simulink model "model_5LinkWalk_NODS_soft_ground"  (R2022b)
settings: Solver=VariableStepAuto  StartTime=0.0  StopTime=Tf  FixedStep=1e-5  MaxStep=1e-3  RelTol=1e-12  AbsTol=1e-8
values from neighbouring files (symbols this model uses):
  gains = [K_p,K_d,K_p,K_d,K_p,K_d,K_p,K_d,K_p,K_d]    [main_soft_ground.m]
  init_flag = [-1; 0; ocl_traj.x_sw(1); init_t_mode_change; alpha_ref(1); 0; y_g_curr]    [main_soft_ground.m]
  Initial_state = [q0;dq0]    [main_soft_ground.m]
  joint_angles_ref = [ocl_traj.time, ocl_traj.simout, alpha_ref]    [main_soft_ground.m]
  landing_ref = [landing_traj.time, landing_traj.simout, alpha_ref_landing]    [main_soft_ground.m]
  param = [ ... (first row only)    [main_soft_ground.m]
  sample_time = time(2) - time(1)    [animation_floating.m]    (also in main_soft_ground.m = 0.001)
undefined symbols (not defined in the file or in its folder): uneven_terrain
libraries: simulink x2
(part 1 of 2)
settings Model: SimulationMode=accelerator  VariantFading=off  Creator=yamakita_lab  LastModifiedBy=mmpel
settings SolverCC: AutoScaleAbsTol=off  AlgebraicLoopSolver=TrustRegion
settings DataIOCC: ReturnWorkspaceOutputs=off
settings DebuggingCC: ParameterPrecisionLossMsg=none  UnconnectedInputMsg=warning  UnconnectedOutputMsg=warning  UnconnectedLineMsg=warning  SFMachineParentedDataDiag=warning  ArithmeticOperatorsInVariantConditions=warning
settings ModelReferenceCC: EnableRefExpFcnMdlSchedulingChecks=on
settings SFSimCC: SimUseLocalCustomCode=off  CustomCodeUndefinedFunction=UseInterfaceOnly
settings RTWCC: RTWUseLocalCustomCode=off  DLArmComputeVersion=19.05

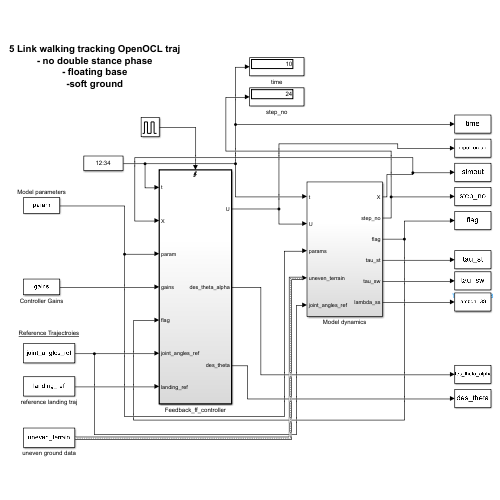
[thumbnail: Simulink's stored preview of the top-level diagram]
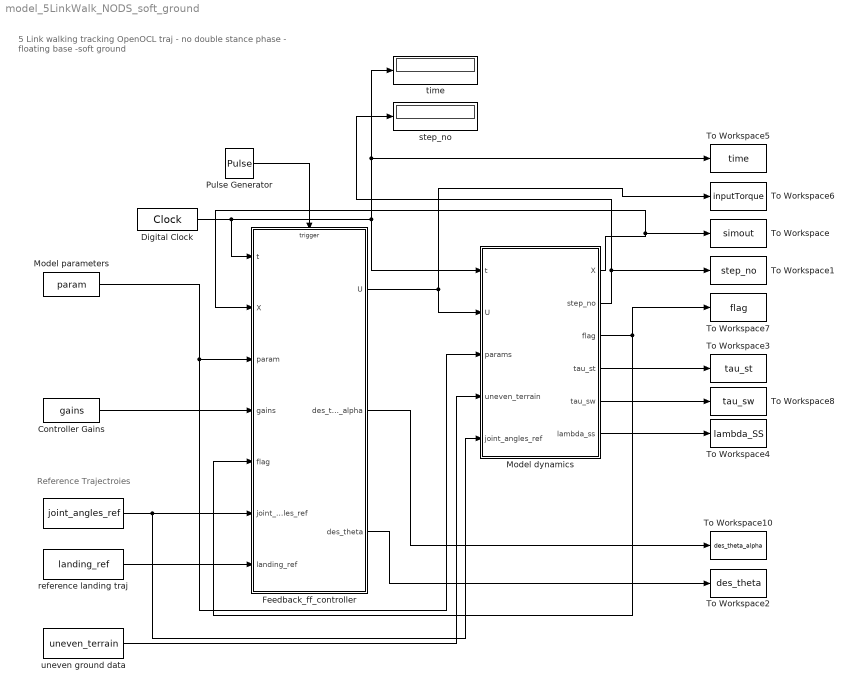
== system model_5LinkWalk_NODS_soft_ground ==
  note: Reference Trajectroies
  note: 5 Link walking tracking OpenOCL traj
      | - no double stance phase
      | - floating base
      | -soft ground
  " " : Constant  Value=joint_angles_ref
  Controller Gains : Constant  Value=gains
  Digital Clock : DigitalClock  SampleTime=1e-4
  Feedback_ff_controller : Subsystem  TreatAsAtomicUnit=on
  Model dynamics : Subsystem
  Model parameters : Constant  Value=param  OutDataTypeStr=double
  Pulse Generator : DiscretePulseGenerator  PulseType=Time based  Period=5e-4  PulseWidth=5
  To Workspace : ToWorkspace  VariableName=simout  SampleTime=sample_time
  To Workspace1 : ToWorkspace  VariableName=step_no  SampleTime=sample_time
  To Workspace10 : ToWorkspace  VariableName=des_theta_alpha  SampleTime=sample_time
  To Workspace2 : ToWorkspace  VariableName=des_theta  SampleTime=sample_time
  To Workspace3 : ToWorkspace  VariableName=tau_st  SampleTime=sample_time
  To Workspace4 : ToWorkspace  VariableName=lambda_SS  SampleTime=sample_time
  To Workspace5 : ToWorkspace  VariableName=time  SampleTime=sample_time
  To Workspace6 : ToWorkspace  VariableName=inputTorque  SampleTime=sample_time
  To Workspace7 : ToWorkspace  VariableName=flag  SampleTime=sample_time
  To Workspace8 : ToWorkspace  VariableName=tau_sw  SampleTime=sample_time
  reference landing traj : Constant  Value=landing_ref
  step_no : Display
  time : Display
  uneven ground data : Constant  Value=uneven_terrain  OutDataTypeStr=Bus: uneven_terrain_bus
  wires:
  Feedback_ff_controller/1(U) -> Model dynamics/2(U), To Workspace6/1
  Model dynamics/1(X) -> To Workspace/1, Feedback_ff_controller/2(X)
  Digital Clock/1 -> time/1, To Workspace5/1, Model dynamics/1(t), Feedback_ff_controller/1(t)
  Model dynamics/2(step_no) -> step_no/1, To Workspace1/1
  Model parameters/1 -> Model dynamics/3(params), Feedback_ff_controller/3(param)
  Controller Gains/1 -> Feedback_ff_controller/4(gains)
  Model dynamics/3(flag) -> Feedback_ff_controller/5(flag), To Workspace7/1
  " "/1 -> Model dynamics/5(joint_angles_ref), Feedback_ff_controller/6(joint_angles_ref)
  Pulse Generator/1 -> Feedback_ff_controller/Trigger
  Model dynamics/4(tau_st) -> To Workspace3/1
  Model dynamics/5(tau_sw) -> To Workspace8/1
  Feedback_ff_controller/2(des_theta_alpha) -> To Workspace10/1
  Feedback_ff_controller/3(des_theta) -> To Workspace2/1
  uneven ground data/1 -> Model dynamics/4(uneven_terrain)
  reference landing traj/1 -> Feedback_ff_controller/7(landing_ref)
  Model dynamics/6(lambda_ss) -> To Workspace4/1

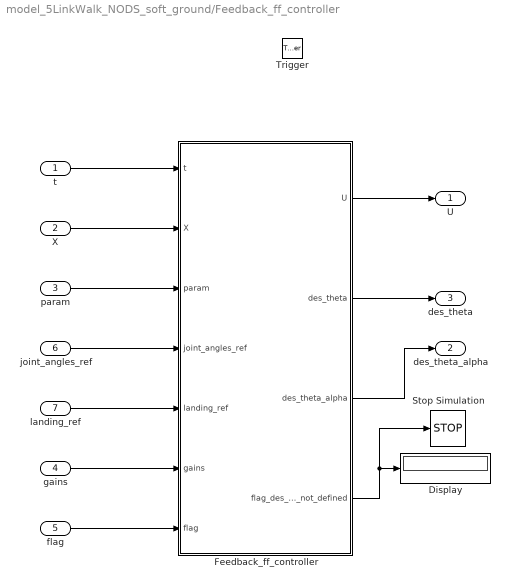
== system model_5LinkWalk_NODS_soft_ground/Feedback_ff_controller ==
  t : Inport
  X : Inport  Port=2
  param : Inport  Port=3
  gains : Inport  Port=4
  flag : Inport  Port=5
  joint_angles_ref : Inport  Port=6
  landing_ref : Inport  Port=7
  Trigger : TriggerPort  VariantControl=Variant  PortDimensions=1
  Display : Display
  Feedback_ff_controller : MATLAB Function  TreatAsAtomicUnit=on
  Stop Simulation : Stop
  U : Outport  VectorParamsAs1DForOutWhenUnconnected=off
  des_theta_alpha : Outport  Port=2  InitialOutput=[0;0;0;0;0; 0;0;0;0;0; 0]  VectorParamsAs1DForOutWhenUnconnected=off
  des_theta : Outport  Port=3  InitialOutput=[0;0;0;0;0; 0;0;0;0;0]  VectorParamsAs1DForOutWhenUnconnected=off
  wires:
  Feedback_ff_controller/1(U) -> U/1
  t/1 -> Feedback_ff_controller/1(t)
  X/1 -> Feedback_ff_controller/2(X)
  param/1 -> Feedback_ff_controller/3(param)
  gains/1 -> Feedback_ff_controller/6(gains)
  flag/1 -> Feedback_ff_controller/7(flag)
  joint_angles_ref/1 -> Feedback_ff_controller/4(joint_angles_ref)
  Feedback_ff_controller/3(des_theta_alpha) -> des_theta_alpha/1
  landing_ref/1 -> Feedback_ff_controller/5(landing_ref)
  Feedback_ff_controller/4(flag_des_theta_not_defined) -> Stop Simulation/1, Display/1
  Feedback_ff_controller/2(des_theta) -> des_theta/1

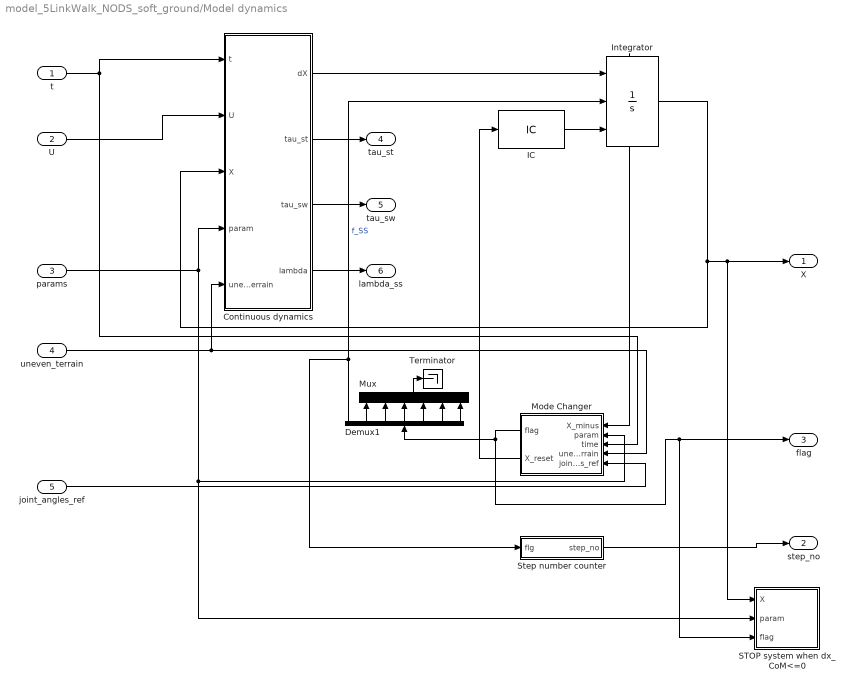
== system model_5LinkWalk_NODS_soft_ground/Model dynamics ==
  t : Inport
  U : Inport  Port=2
  params : Inport  Port=3
  uneven_terrain : Inport  Port=4
  joint_angles_ref : Inport  Port=5
  Continuous dynamics : MATLAB Function  TreatAsAtomicUnit=on
  Demux1 : Demux  Outputs=7
  IC : InitialCondition  Value=Initial_state
  Integrator : Integrator  ExternalReset=rising  InitialConditionSource=external  ShowStatePort=on
  Mode Changer : Subsystem
  Mux : Mux  Inputs=6
  STOP system when dx_CoM<=0 : Subsystem
  Step number counter : Subsystem
  Terminator : Terminator
  X : Outport  VectorParamsAs1DForOutWhenUnconnected=off
  step_no : Outport  Port=2  VectorParamsAs1DForOutWhenUnconnected=off
  flag : Outport  Port=3
  tau_st : Outport  Port=4  VectorParamsAs1DForOutWhenUnconnected=off
  tau_sw : Outport  Port=5  VectorParamsAs1DForOutWhenUnconnected=off
  lambda_ss : Outport  Port=6  VectorParamsAs1DForOutWhenUnconnected=off
  wires:
  IC/1 -> Integrator/3
  Integrator/State -> Mode Changer/1(X_minus)
  Continuous dynamics/1(dX) -> Integrator/1
  params/1 -> Continuous dynamics/4(param), STOP system when dx_CoM<=0/2(param), Mode Changer/2("param ")
  U/1 -> Continuous dynamics/2(U)
  t/1 -> Continuous dynamics/1(t), Mode Changer/3(time)
  Integrator/1 -> STOP system when dx_CoM<=0/1(X), X/1, Continuous dynamics/3(X)
  Mode Changer/2(X_reset) -> IC/1
  Mode Changer/1(flag) -> STOP system when dx_CoM<=0/3(flag), flag/1, Demux1/1
  Demux1/1 -> Integrator/2, Step number counter/1(flg)  "f_SS"
  Step number counter/1(step_no) -> step_no/1
  Continuous dynamics/2(tau_st) -> tau_st/1
  Continuous dynamics/3(tau_sw) -> tau_sw/1
  Demux1/2 -> Mux/1
  Demux1/3 -> Mux/2
  Demux1/4 -> Mux/3
  Demux1/5 -> Mux/4
  Demux1/6 -> Mux/5
  Mux/1 -> Terminator/1
  uneven_terrain/1 -> Continuous dynamics/5(uneven_terrain), Mode Changer/4(uneven_terrain)
  Demux1/7 -> Mux/6
  joint_angles_ref/1 -> Mode Changer/5(joint_angles_ref)
  Continuous dynamics/4(lambda) -> lambda_ss/1

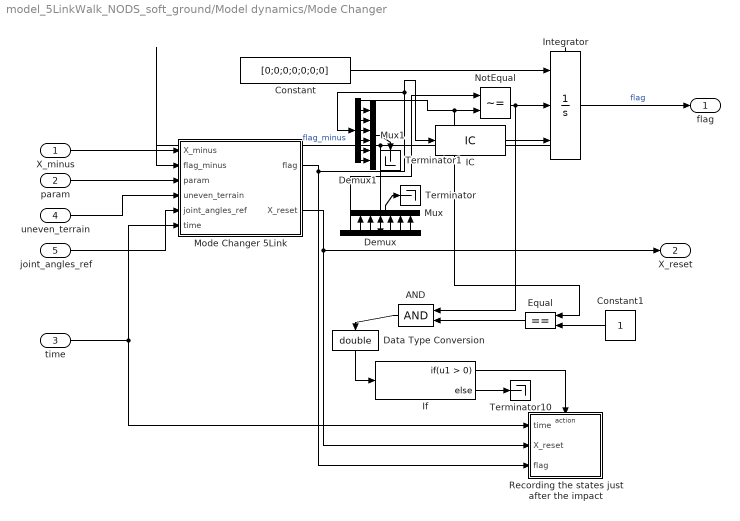
== system model_5LinkWalk_NODS_soft_ground/Model dynamics/Mode Changer ==
  X_minus : Inport
  "param " : Inport  Port=2
  time : Inport  Port=3
  uneven_terrain : Inport  Port=4
  joint_angles_ref : Inport  Port=5
  AND : Logic  IconShape=distinctive  AllPortsSameDT=off  OutDataTypeStr=boolean
  Constant : Constant  Value=[0;0;0;0;0;0;0]
  Constant1 : Constant
  Data Type Conversion : DataTypeConversion  OutDataTypeStr=double  SaturateOnIntegerOverflow=off  RndMeth=Floor
  Demux : Demux  Outputs=7
  Demux1 : Demux  Outputs=7
  Equal : RelationalOperator  Operator===  OutDataTypeStr=boolean  RndMeth=Simplest  InputSameDT=off
  IC : InitialCondition  Value=init_flag
  If : If
  Integrator : Integrator  ExternalReset=rising  InitialConditionSource=external  ShowStatePort=on
  Mode Changer 5Link : MATLAB Function  TreatAsAtomicUnit=on
  Mux : Mux  Inputs=6
  Mux1 : Mux  Inputs=6
  NotEqual : RelationalOperator  Operator=~=  OutDataTypeStr=boolean  RndMeth=Simplest  InputSameDT=off
  Recording the states just after the impact : Subsystem  TreatAsAtomicUnit=on
  Terminator : Terminator
  Terminator1 : Terminator
  Terminator10 : Terminator
  flag : Outport  VectorParamsAs1DForOutWhenUnconnected=off
  X_reset : Outport  Port=2  VectorParamsAs1DForOutWhenUnconnected=off
  wires:
  X_minus/1 -> Mode Changer 5Link/1(X_minus)
  IC/1 -> Integrator/3
  Integrator/State -> Mode Changer 5Link/2(flag_minus), Demux/1  "flag_minus"
  "param "/1 -> Mode Changer 5Link/3(param)
  Mode Changer 5Link/1(flag) -> Demux1/1, IC/1, Recording the states just after the impact/3(flag)
  Constant/1 -> Integrator/1
  NotEqual/1 -> AND/1, Integrator/2
  Integrator/1 -> flag/1  "flag"
  Mode Changer 5Link/2(X_reset) -> Recording the states just after the impact/2(X_reset), X_reset/1
  Demux/1 -> NotEqual/1
  time/1 -> Mode Changer 5Link/6(time), Recording the states just after the impact/1(time)
  Demux1/1 -> Equal/1, NotEqual/2
  If/1 -> Recording the states just after the impact/Action
  If/2 -> Terminator10/1
  Data Type Conversion/1 -> If/1
  AND/1 -> Data Type Conversion/1
  Equal/1 -> AND/2
  Constant1/1 -> Equal/2
  uneven_terrain/1 -> Mode Changer 5Link/4(uneven_terrain)
  Demux/2 -> Mux/1
  Demux/3 -> Mux/2
  Demux/4 -> Mux/3
  Demux/5 -> Mux/4
  Demux/6 -> Mux/5
  Demux/7 -> Mux/6
  Mux/1 -> Terminator/1
  Demux1/2 -> Mux1/1
  Demux1/3 -> Mux1/2
  Demux1/4 -> Mux1/3
  Demux1/5 -> Mux1/4
  Demux1/6 -> Mux1/5
  Demux1/7 -> Mux1/6
  Mux1/1 -> Terminator1/1
  joint_angles_ref/1 -> Mode Changer 5Link/5(joint_angles_ref)

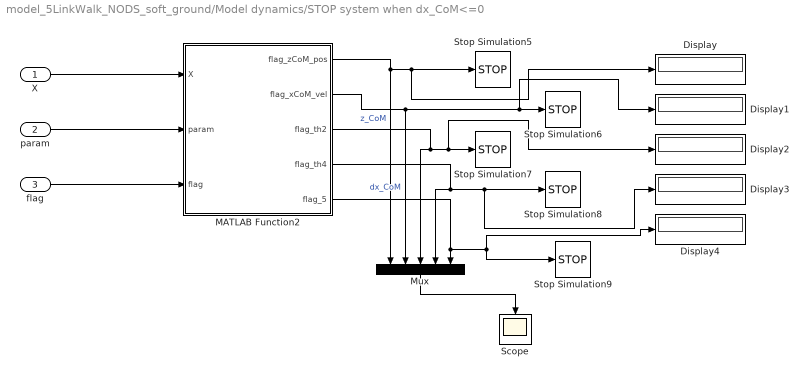
== system model_5LinkWalk_NODS_soft_ground/Model dynamics/STOP system when dx_CoM<=0 ==
  X : Inport
  param : Inport  Port=2
  flag : Inport  Port=3
  Display{,1..4} (5 alike) : Display
  MATLAB Function2 : MATLAB Function  TreatAsAtomicUnit=on
  Mux : Mux  Inputs=5
  Scope : Scope
  Stop Simulation{5..9} (5 alike) : Stop
  wires:
  X/1 -> MATLAB Function2/1(X)
  param/1 -> MATLAB Function2/2(param)
  flag/1 -> MATLAB Function2/3(flag)
  MATLAB Function2/1(flag_zCoM_pos) -> Mux/1, Display/1, Stop Simulation5/1  "z_CoM"
  MATLAB Function2/2(flag_xCoM_vel) -> Display1/1, Stop Simulation6/1, Mux/2  "dx_CoM"
  MATLAB Function2/4(flag_th4) -> Mux/4, Display3/1, Stop Simulation8/1
  Mux/1 -> Scope/1
  MATLAB Function2/3(flag_th2) -> Display2/1, Stop Simulation7/1, Mux/3
  MATLAB Function2/5(flag_5) -> Display4/1, Stop Simulation9/1, Mux/5

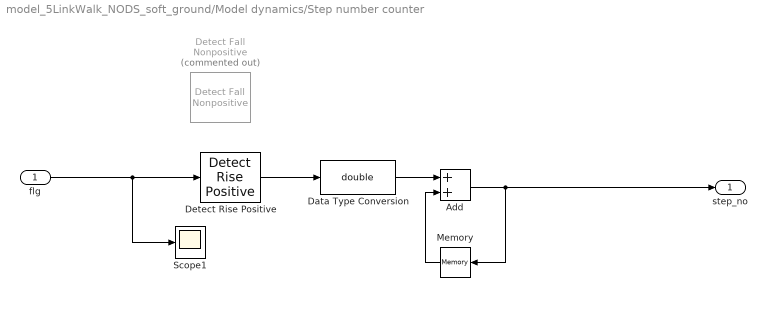
== system model_5LinkWalk_NODS_soft_ground/Model dynamics/Step number counter ==
  flg : Inport  SampleTime=sample_time
  Add : Sum
  Data Type Conversion : DataTypeConversion  OutDataTypeStr=double  SaturateOnIntegerOverflow=off  RndMeth=Floor
  Detect Fall Nonpositive : simulink/Logic and Bit Operations/Detect Fall Nonpositive  Commented=on  vinit=1  OutDataTypeStr=boolean
  Detect Rise Positive : simulink/Logic and Bit Operations/Detect Rise Positive  vinit=-1  OutDataTypeStr=boolean
  Memory : Memory  InheritSampleTime=on
  Scope1 : Scope
  step_no : Outport  VectorParamsAs1DForOutWhenUnconnected=off
  wires:
  Add/1 -> step_no/1, Memory/1
  Memory/1 -> Add/2
  flg/1 -> Detect Rise Positive/1, Scope1/1
  Data Type Conversion/1 -> Add/1
  Detect Rise Positive/1 -> Data Type Conversion/1

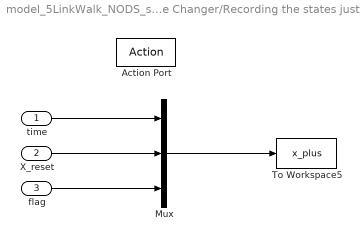
== system model_5LinkWalk_NODS_soft_ground/Model dynamics/Mode Changer/Recording the states just after the impact ==
  time : Inport
  X_reset : Inport  Port=2
  flag : Inport  Port=3
  Action Port : ActionPort  ActionPortLabel=if(u1 > 0)
  Mux : Mux  Inputs=3
  To Workspace5 : ToWorkspace  VariableName=x_plus  SampleTime=-1
  wires:
  time/1 -> Mux/1
  X_reset/1 -> Mux/2
  flag/1 -> Mux/3
  Mux/1 -> To Workspace5/1

== matlab function model_5LinkWalk_NODS_soft_ground/Model dynamics/Continuous dynamics ==
  data: t input; U input; dX output; X input; param input; tau_st output; tau_sw output; lambda output; uneven_terrain input
function [dX, tau_st, tau_sw, lambda] = fcn(t, U, X, param, uneven_terrain)

%% variables
x_st = X(1);
y_st = X(2);
th1 = X(3);
th2 = X(4);
th3 = X(5);
th4 = X(6);
th5 = X(7);

dx_st = X(8);
dy_st = X(9);
dth1 = X(10);
dth2 = X(11);
dth3 = X(12);
dth4 = X(13);
dth5 = X(14);

q = [x_st; y_st; th1; th2; th3; th4; th5];
dq = [dx_st; dy_st; dth1; dth2; dth3; dth4; dth5];

%% parameters

m1 = param(1);
m2 = param(2);
m3 = m2;
m4 = m1;
m5 = param(3);

l1 = param(4);
l2 = param(5);
l5 = param(6);
l3 = l2;
l4 = l1;

gravi = param(7);
I1 = param(8);
I2 = param(9);
I5 = param(10);
I3 = I1;
I4 = I2;

r_k = param(11);
r_h = param(12);
k_ba = param(13);
phi_h0 = param(14);
phi_k0 = param(15);

% ground parameters
k_ground = param(16);
d_ground = param(17);

%% ground height below the stance foot
x_ground = uneven_terrain.track_start:uneven_terrain.dist_step_size:uneven_terrain.track_end;
y_ground = uneven_terrain.y_g_curr;
y_ground_curr = interp1(x_ground, y_ground, x_st);

%% flags
% f_SS = flag(1); % indicates which stance phase it is
% foot = flag(2); % location of the stance foot
% foot_prev = flag(3); % previous location of the stance foot

%% Inertia Matrix
MM = [m1 + m2 + m3 + m4 + m5, 0, - (m3*(2*l2*sin(th1 + th2) + 2*l1*sin(th1) + l3*sin(th1 + th2 + th3)))/2 - (m5*(2*l2*sin(th1 + th2) + 2*l1*sin(th1) + l5*sin(th1 + th2 + th5)))/2 - (m2*(l2*sin(th1 + th2) + 2*l1*sin(th1)))/2 - (m4*(l4*sin(th1 + th2 + th3 + th4) + 2*l2*sin(th1 + th2) + 2*l1*sin(th1) + 2*l3*sin(th1 + th2 + th3)))/2 - (l1*m1*sin(th1))/2, - (m4*(l4*sin(th1 + th2 + th3 + th4) + 2*l2*sin(th1 + th2) + 2*l3*sin(th1 + th2 + th3)))/2 - (m3*(2*l2*sin(th1 + th2) + l3*sin(th1 + th2 + th3)))/2 - (m5*(2*l2*sin(th1 + th2) + l5*sin(th1 + th2 + th5)))/2 - (l2*m2*sin(th1 + th2))/2, - (m4*(l4*sin(th1 + th2 + th3 + th4) + 2*l3*sin(th1 + th2 + th3)))/2 - (l3*m3*sin(th1 + th2 + th3))/2, -(l4*m4*sin(th1 + th2 + th3 + th4))/2, -(l5*m5*sin(th1 + th2 + th5))/2; 0, m1 + m2 + m3 + m4 + m5, (m3*(2*l2*cos(th1 + th2) + 2*l1*cos(th1) + l3*cos(th1 + th2 + th3)))/2 + (m5*(2*l2*cos(th1 + th2) + 2*l1*cos(th1) + l5*cos(th1 + th2 + th5)))/2 + (m2*(l2*cos(th1 + th2) + 2*l1*cos(th1)))/2 + (m4*(l4*cos(th1 + th2 + th3 + th4) + 2*l2*cos(th1 + th2) + 2*l1*cos(th1) + 2*l3*cos(th1 + th2 + th3)))/2 + (l1*m1*cos(th1))/2, (m3*(2*l2*cos(th1 + th2) + l3*cos(th1 + th2 + th3)))/2 + (m5*(2*l2*cos(th1 + th2) + l5*cos(th1 + th2 + th5)))/2 + (m4*(l4*cos(th1 + th2 + th3 + th4) + 2*l2*cos(th1 + th2) + 2*l3*cos(th1 + th2 + th3)))/2 + (l2*m2*cos(th1 + th2))/2, (m4*(l4*cos(th1 + th2 + th3 + th4) + 2*l3*cos(th1 + th2 + th3)))/2 + (l3*m3*cos(th1 + th2 + th3))/2, (l4*m4*cos(th1 + th2 + th3 + th4))/2, (l5*m5*cos(th1 + th2 + th5))/2; - (m3*(2*l2*sin(th1 + th2) + 2*l1*sin(th1) + l3*sin(th1 + th2 + th3)))/2 - (m5*(2*l2*sin(th1 + th2) + 2*l1*sin(th1) + l5*sin(th1 + th2 + th5)))/2 - (m2*(l2*sin(th1 + th2) + 2*l1*sin(th1)))/2 - (m4*(l4*sin(th1 + th2 + th3 + th4) + 2*l2*sin(th1 + th2) + 2*l1*sin(th1) + 2*l3*sin(th1 + th2 + th3)))/2 - (l1*m1*sin(th1))/2, (m3*(2*l2*cos(th1 + th2) + 2*l1*cos(th1) + l3*cos(th1 + th2 + th3)))/2 + (m5*(2*l2*cos(th1 + th2) + 2*l1*cos(th1) + l5*cos(th1 + th2 + th5)))/2 + (m2*(l2*cos(th1 + th2) + 2*l1*cos(th1)))/2 + (m4*(l4*cos(th1 + th2 + th3 + th4) + 2*l2*cos(th1 + th2) + 2*l1*cos(th1) + 2*l3*cos(th1 + th2 + th3)))/2 + (l1*m1*cos(th1))/2, I1 + I2 + I3 + I4 + I5 + (l1^2*m1)/4 + l1^2*m2 + l1^2*m3 + (l2^2*m2)/4 + l1^2*m4 + l2^2*m3 + l1^2*m5 + l2^2*m4 + (l3^2*m3)/4 + l2^2*m5 + l3^2*m4 + (l4^2*m4)/4 + (l5^2*m5)/4 + l1*l3*m3*cos(th2 + th3) + 2*l1*l3*m4*cos(th2 + th3) + l2*l4*m4*cos(th3 + th4) + l1*l5*m5*cos(th2 + th5) + l1*l2*m2*cos(th2) + 2*l1*l2*m3*cos(th2) + 2*l1*l2*m4*cos(th2) + 2*l1*l2*m5*cos(th2) + l2*l3*m3*cos(th3) + 2*l2*l3*m4*cos(th3) + l3*l4*m4*cos(th4) + l2*l5*m5*cos(th5) + l1*l4*m4*cos(th2 + th3 + th4), I2 + I3 + I4 + I5 + (l2^2*m2)/4 + l2^2*m3 + l2^2*m4 + (l3^2*m3)/4 + l2^2*m5 + l3^2*m4 + (l4^2*m4)/4 + (l5^2*m5)/4 + (l1*l3*m3*cos(th2 + th3))/2 + l1*l3*m4*cos(th2 + th3) + l2*l4*m4*cos(th3 + th4) + (l1*l5*m5*cos(th2 + th5))/2 + (l1*l2*m2*cos(th2))/2 + l1*l2*m3*cos(th2) + l1*l2*m4*cos(th2) + l1*l2*m5*cos(th2) + l2*l3*m3*cos(th3) + 2*l2*l3*m4*cos(th3) + l3*l4*m4*cos(th4) + l2*l5*m5*cos(th5) + (l1*l4*m4*cos(th2 + th3 + th4))/2, I3 + I4 + (l3^2*m3)/4 + l3^2*m4 + (l4^2*m4)/4 + (l1*l3*m3*cos(th2 + th3))/2 + l1*l3*m4*cos(th2 + th3) + (l2*l4*m4*cos(th3 + th4))/2 + (l2*l3*m3*cos(th3))/2 + l2*l3*m4*cos(th3) + l3*l4*m4*cos(th4) + (l1*l4*m4*cos(th2 + th3 + th4))/2, I4 + (l4^2*m4)/4 + (l2*l4*m4*cos(th3 + th4))/2 + (l3*l4*m4*cos(th4))/2 + (l1*l4*m4*cos(th2 + th3 + th4))/2, I5 + (l5^2*m5)/4 + (l1*l5*m5*cos(th2 + th5))/2 + (l2*l5*m5*cos(th5))/2; - (m4*(l4*sin(th1 + th2 + th3 + th4) + 2*l2*sin(th1 + th2) + 2*l3*sin(th1 + th2 + th3)))/2 - (m3*(2*l2*sin(th1 + th2) + l3*sin(th1 + th2 + th3)))/2 - (m5*(2*l2*sin(th1 + th2) + l5*sin(th1 + th2 + th5)))/2 - (l2*m2*sin(th1 + th2))/2, (m3*(2*l2*cos(th1 + th2) + l3*cos(th1 + th2 + th3)))/2 + (m5*(2*l2*cos(th1 + th2) + l5*cos(th1 + th2 + th5)))/2 + (m4*(l4*cos(th1 + th2 + th3 + th4) + 2*l2*cos(th1 + th2) + 2*l3*cos(th1 + th2 + th3)))/2 + (l2*m2*cos(th1 + th2))/2, I2 + I3 + I4 + I5 + (l2^2*m2)/4 + l2^2*m3 + l2^2*m4 + (l3^2*m3)/4 + l2^2*m5 + l3^2*m4 + (l4^2*m4)/4 + (l5^2*m5)/4 + (l1*l3*m3*cos(th2 + th3))/2 + l1*l3*m4*cos(th2 + th3) + l2*l4*m4*cos(th3 + th4) + (l1*l5*m5*cos(th2 + th5))/2 + (l1*l2*m2*cos(th2))/2 + l1*l2*m3*cos(th2) + l1*l2*m4*cos(th2) + l1*l2*m5*cos(th2) + l2*l3*m3*cos(th3) + 2*l2*l3*m4*cos(th3) + l3*l4*m4*cos(th4) + l2*l5*m5*cos(th5) + (l1*l4*m4*cos(th2 + th3 + th4))/2, I2 + I3 + I4 + I5 + (l2^2*m2)/4 + l2^2*m3 + l2^2*m4 + (l3^2*m3)/4 + l2^2*m5 + l3^2*m4 + (l4^2*m4)/4 + (l5^2*m5)/4 + l2*l4*m4*cos(th3 + th4) + l2*l3*m3*cos(th3) + 2*l2*l3*m4*cos(th3) + l3*l4*m4*cos(th4) + l2*l5*m5*cos(th5), I3 + I4 + (l3^2*m3)/4 + l3^2*m4 + (l4^2*m4)/4 + (l2*l4*m4*cos(th3 + th4))/2 + (l2*l3*m3*cos(th3))/2 + l2*l3*m4*cos(th3) + l3*l4*m4*cos(th4), I4 + (l4^2*m4)/4 + (l2*l4*m4*cos(th3 + th4))/2 + (l3*l4*m4*cos(th4))/2, I5 + (l5^2*m5)/4 + (l2*l5*m5*cos(th5))/2; - (m4*(l4*sin(th1 + th2 + th3 + th4) + 2*l3*sin(th1 + th2 + th3)))/2 - (l3*m3*sin(th1 + th2 + th3))/2, (m4*(l4*cos(th1 + th2 + th3 + th4) + 2*l3*cos(th1 + th2 + th3)))/2 + (l3*m3*cos(th1 + th2 + th3))/2, I3 + I4 + (l3^2*m3)/4 + l3^2*m4 + (l4^2*m4)/4 + (l1*l3*m3*cos(th2 + th3))/2 + l1*l3*m4*cos(th2 + th3) + (l2*l4*m4*cos(th3 + th4))/2 + (l2*l3*m3*cos(th3))/2 + l2*l3*m4*cos(th3) + l3*l4*m4*cos(th4) + (l1*l4*m4*cos(th2 + th3 + th4))/2, I3 + I4 + (l3^2*m3)/4 + l3^2*m4 + (l4^2*m4)/4 + (l2*l4*m4*cos(th3 + th4))/2 + (l2*l3*m3*cos(th3))/2 + l2*l3*m4*cos(th3) + l3*l4*m4*cos(th4), I3 + I4 + (l3^2*m3)/4 + l3^2*m4 + (l4^2*m4)/4 + l3*l4*m4*cos(th4), I4 + (l4^2*m4)/4 + (l3*l4*m4*cos(th4))/2, 0; -(l4*m4*sin(th1 + th2 + th3 + th4))/2, (l4*m4*cos(th1 + th2 + th3 + th4))/2, I4 + (l4^2*m4)/4 + (l2*l4*m4*cos(th3 + th4))/2 + (l3*l4*m4*cos(th4))/2 + (l1*l4*m4*cos(th2 + th3 + th4))/2, I4 + (l4^2*m4)/4 + (l2*l4*m4*cos(th3 + th4))/2 + (l3*l4*m4*cos(th4))/2, I4 + (l4^2*m4)/4 + (l3*l4*m4*cos(th4))/2, I4 + (l4^2*m4)/4, 0; -(l5*m5*sin(th1 + th2 + th5))/2, (l5*m5*cos(th1 + th2 + th5))/2, I5 + (l5^2*m5)/4 + (l1*l5*m5*cos(th2 + th5))/2 + (l2*l5*m5*cos(th5))/2, I5 + (l5^2*m5)/4 + (l2*l5*m5*cos(th5))/2, 0, 0, I5 + (l5^2*m5)/4];

%% Coriolis, centrifugal and gravity terms
HH = [- (dth1^2*l3*m3*cos(th1 + th2 + th3))/2 - dth1^2*l3*m4*cos(th1 + th2 + th3) - (dth2^2*l3*m3*cos(th1 + th2 + th3))/2 - dth2^2*l3*m4*cos(th1 + th2 + th3) - (dth3^2*l3*m3*cos(th1 + th2 + th3))/2 - dth3^2*l3*m4*cos(th1 + th2 + th3) - (dth1^2*l5*m5*cos(th1 + th2 + th5))/2 - (dth2^2*l5*m5*cos(th1 + th2 + th5))/2 - (dth5^2*l5*m5*cos(th1 + th2 + th5))/2 - (dth1^2*l4*m4*cos(th1 + th2 + th3 + th4))/2 - (dth2^2*l4*m4*cos(th1 + th2 + th3 + th4))/2 - (dth3^2*l4*m4*cos(th1 + th2 + th3 + th4))/2 - (dth4^2*l4*m4*cos(th1 + th2 + th3 + th4))/2 - (dth1^2*l2*m2*cos(th1 + th2))/2 - dth1^2*l2*m3*cos(th1 + th2) - (dth2^2*l2*m2*cos(th1 + th2))/2 - dth1^2*l2*m4*cos(th1 + th2) - dth2^2*l2*m3*cos(th1 + th2) - dth1^2*l2*m5*cos(th1 + th2) - dth2^2*l2*m4*cos(th1 + th2) - dth2^2*l2*m5*cos(th1 + th2) - (dth1^2*l1*m1*cos(th1))/2 - dth1^2*l1*m2*cos(th1) - dth1^2*l1*m3*cos(th1) - dth1^2*l1*m4*cos(th1) - dth1^2*l1*m5*cos(th1) - dth1*dth2*l3*m3*cos(th1 + th2 + th3) - 2*dth1*dth2*l3*m4*cos(th1 + th2 + th3) - dth1*dth3*l3*m3*cos(th1 + th2 + th3) - 2*dth1*dth3*l3*m4*cos(th1 + th2 + th3) - dth2*dth3*l3*m3*cos(th1 + th2 + th3) - 2*dth2*dth3*l3*m4*cos(th1 + th2 + th3) - dth1*dth2*l5*m5*cos(th1 + th2 + th5) - dth1*dth5*l5*m5*cos(th1 + th2 + th5) - dth2*dth5*l5*m5*cos(th1 + th2 + th5) - dth1*dth2*l4*m4*cos(th1 + th2 + th3 + th4) - dth1*dth3*l4*m4*cos(th1 + th2 + th3 + th4) - dth1*dth4*l4*m4*cos(th1 + th2 + th3 + th4) - dth2*dth3*l4*m4*cos(th1 + th2 + th3 + th4) - dth2*dth4*l4*m4*cos(th1 + th2 + th3 + th4) - dth3*dth4*l4*m4*cos(th1 + th2 + th3 + th4) - dth1*dth2*l2*m2*cos(th1 + th2) - 2*dth1*dth2*l2*m3*cos(th1 + th2) - 2*dth1*dth2*l2*m4*cos(th1 + th2) - 2*dth1*dth2*l2*m5*cos(th1 + th2); (m1 + m2 + m3 + m4 + m5)*gravi - (dth1^2*l3*m3*sin(th1 + th2 + th3))/2 - dth1^2*l3*m4*sin(th1 + th2 + th3) - (dth2^2*l3*m3*sin(th1 + th2 + th3))/2 - dth2^2*l3*m4*sin(th1 + th2 + th3) - (dth3^2*l3*m3*sin(th1 + th2 + th3))/2 - dth3^2*l3*m4*sin(th1 + th2 + th3) - (dth1^2*l5*m5*sin(th1 + th2 + th5))/2 - (dth2^2*l5*m5*sin(th1 + th2 + th5))/2 - (dth5^2*l5*m5*sin(th1 + th2 + th5))/2 - (dth1^2*l4*m4*sin(th1 + th2 + th3 + th4))/2 - (dth2^2*l4*m4*sin(th1 + th2 + th3 + th4))/2 - (dth3^2*l4*m4*sin(th1 + th2 + th3 + th4))/2 - (dth4^2*l4*m4*sin(th1 + th2 + th3 + th4))/2 - (dth1^2*l2*m2*sin(th1 + th2))/2 - dth1^2*l2*m3*sin(th1 + th2) - (dth2^2*l2*m2*sin(th1 + th2))/2 - dth1^2*l2*m4*sin(th1 + th2) - dth2^2*l2*m3*sin(th1 + th2) - dth1^2*l2*m5*sin(th1 + th2) - dth2^2*l2*m4*sin(th1 + th2) - dth2^2*l2*m5*sin(th1 + th2) - (dth1^2*l1*m1*sin(th1))/2 - dth1^2*l1*m2*sin(th1) - dth1^2*l1*m3*sin(th1) - dth1^2*l1*m4*sin(th1) - dth1^2*l1*m5*sin(th1) - dth1*dth2*l3*m3*sin(th1 + th2 + th3) - 2*dth1*dth2*l3*m4*sin(th1 + th2 + th3) - dth1*dth3*l3*m3*sin(th1 + th2 + th3) - 2*dth1*dth3*l3*m4*sin(th1 + th2 + th3) - dth2*dth3*l3*m3*sin(th1 + th2 + th3) - 2*dth2*dth3*l3*m4*sin(th1 + th2 + th3) - dth1*dth2*l5*m5*sin(th1 + th2 + th5) - dth1*dth5*l5*m5*sin(th1 + th2 + th5) - dth2*dth5*l5*m5*sin(th1 + th2 + th5) - dth1*dth2*l4*m4*sin(th1 + th2 + th3 + th4) - dth1*dth3*l4*m4*sin(th1 + th2 + th3 + th4) - dth1*dth4*l4*m4*sin(th1 + th2 + th3 + th4) - dth2*dth3*l4*m4*sin(th1 + th2 + th3 + th4) - dth2*dth4*l4*m4*sin(th1 + th2 + th3 + th4) - dth3*dth4*l4*m4*sin(th1 + th2 + th3 + th4) - dth1*dth2*l2*m2*sin(th1 + th2) - 2*dth1*dth2*l2*m3*sin(th1 + th2) - 2*dth1*dth2*l2*m4*sin(th1 + th2) - 2*dth1*dth2*l2*m5*sin(th1 + th2); (gravi*l4*m4*cos(th1 + th2 + th3 + th4))/2 + (gravi*l2*m2*cos(th1 + th2))/2 + gravi*l2*m3*cos(th1 + th2) + gravi*l2*m4*cos(th1 + th2) + gravi*l2*m5*cos(th1 + th2) + (gravi*l1*m1*cos(th1))/2 + gravi*l1*m2*cos(th1) + gravi*l1*m3*cos(th1) + gravi*l1*m4*cos(th1) + gravi*l1*m5*cos(th1) + (gravi*l3*m3*cos(th1 + th2 + th3))/2 + gravi*l3*m4*cos(th1 + th2 + th3) + (gravi*l5*m5*cos(th1 + th2 + th5))/2 - (dth2^2*l1*l3*m3*sin(th2 + th3))/2 - dth2^2*l1*l3*m4*sin(th2 + th3) - (dth3^2*l1*l3*m3*sin(th2 + th3))/2 - dth3^2*l1*l3*m4*sin(th2 + th3) - (dth2^2*l1*l5*m5*sin(th2 + th5))/2 - (dth3^2*l2*l4*m4*sin(th3 + th4))/2 - (dth4^2*l2*l4*m4*sin(th3 + th4))/2 - (dth5^2*l1*l5*m5*sin(th2 + th5))/2 - (dth2^2*l1*l2*m2*sin(th2))/2 - dth2^2*l1*l2*m3*sin(th2) - dth2^2*l1*l2*m4*sin(th2) - dth2^2*l1*l2*m5*sin(th2) - (dth3^2*l2*l3*m3*sin(th3))/2 - dth3^2*l2*l3*m4*sin(th3) - (dth4^2*l3*l4*m4*sin(th4))/2 - (dth5^2*l2*l5*m5*sin(th5))/2 - (dth2^2*l1*l4*m4*sin(th2 + th3 + th4))/2 - (dth3^2*l1*l4*m4*sin(th2 + th3 + th4))/2 - (dth4^2*l1*l4*m4*sin(th2 + th3 + th4))/2 - dth1*dth2*l1*l3*m3*sin(th2 + th3) - 2*dth1*dth2*l1*l3*m4*sin(th2 + th3) - dth1*dth3*l1*l3*m3*sin(th2 + th3) - 2*dth1*dth3*l1*l3*m4*sin(th2 + th3) - dth2*dth3*l1*l3*m3*sin(th2 + th3) - 2*dth2*dth3*l1*l3*m4*sin(th2 + th3) - dth1*dth2*l1*l5*m5*sin(th2 + th5) - dth1*dth3*l2*l4*m4*sin(th3 + th4) - dth1*dth4*l2*l4*m4*sin(th3 + th4) - dth2*dth3*l2*l4*m4*sin(th3 + th4) - dth2*dth4*l2*l4*m4*sin(th3 + th4) - dth1*dth5*l1*l5*m5*sin(th2 + th5) - dth3*dth4*l2*l4*m4*sin(th3 + th4) - dth2*dth5*l1*l5*m5*sin(th2 + th5) - dth1*dth2*l1*l2*m2*sin(th2) - 2*dth1*dth2*l1*l2*m3*sin(th2) - 2*dth1*dth2*l1*l2*m4*sin(th2) - 2*dth1*dth2*l1*l2*m5*sin(th2) - dth1*dth3*l2*l3*m3*sin(th3) - 2*dth1*dth3*l2*l3*m4*sin(th3) - dth2*dth3*l2*l3*m3*sin(th3) - 2*dth2*dth3*l2*l3*m4*sin(th3) - dth1*dth4*l3*l4*m4*sin(th4) - dth2*dth4*l3*l4*m4*sin(th4) - dth3*dth4*l3*l4*m4*sin(th4) - dth1*dth5*l2*l5*m5*sin(th5) - dth2*dth5*l2*l5*m5*sin(th5) - dth1*dth2*l1*l4*m4*sin(th2 + th3 + th4) - dth1*dth3*l1*l4*m4*sin(th2 + th3 + th4) - dth1*dth4*l1*l4*m4*sin(th2 + th3 + th4) - dth2*dth3*l1*l4*m4*sin(th2 + th3 + th4) - dth2*dth4*l1*l4*m4*sin(th2 + th3 + th4) - dth3*dth4*l1*l4*m4*sin(th2 + th3 + th4); (gravi*l4*m4*cos(th1 + th2 + th3 + th4))/2 + (gravi*l2*m2*cos(th1 + th2))/2 + gravi*l2*m3*cos(th1 + th2) + gravi*l2*m4*cos(th1 + th2) + gravi*l2*m5*cos(th1 + th2) + (gravi*l3*m3*cos(th1 + th2 + th3))/2 + gravi*l3*m4*cos(th1 + th2 + th3) + (gravi*l5*m5*cos(th1 + th2 + th5))/2 + (dth1^2*l1*l3*m3*sin(th2 + th3))/2 + dth1^2*l1*l3*m4*sin(th2 + th3) + (dth1^2*l1*l5*m5*sin(th2 + th5))/2 - (dth3^2*l2*l4*m4*sin(th3 + th4))/2 - (dth4^2*l2*l4*m4*sin(th3 + th4))/2 + (dth1^2*l1*l2*m2*sin(th2))/2 + dth1^2*l1*l2*m3*sin(th2) + dth1^2*l1*l2*m4*sin(th2) + dth1^2*l1*l2*m5*sin(th2) - (dth3^2*l2*l3*m3*sin(th3))/2 - dth3^2*l2*l3*m4*sin(th3) - (dth4^2*l3*l4*m4*sin(th4))/2 - (dth5^2*l2*l5*m5*sin(th5))/2 + (dth1^2*l1*l4*m4*sin(th2 + th3 + th4))/2 - dth1*dth3*l2*l4*m4*sin(th3 + th4) - dth1*dth4*l2*l4*m4*sin(th3 + th4) - dth2*dth3*l2*l4*m4*sin(th3 + th4) - dth2*dth4*l2*l4*m4*sin(th3 + th4) - dth3*dth4*l2*l4*m4*sin(th3 + th4) - dth1*dth3*l2*l3*m3*sin(th3) - 2*dth1*dth3*l2*l3*m4*sin(th3) - dth2*dth3*l2*l3*m3*sin(th3) - 2*dth2*dth3*l2*l3*m4*sin(th3) - dth1*dth4*l3*l4*m4*sin(th4) - dth2*dth4*l3*l4*m4*sin(th4) - dth3*dth4*l3*l4*m4*sin(th4) - dth1*dth5*l2*l5*m5*sin(th5) - dth2*dth5*l2*l5*m5*sin(th5); (gravi*l4*m4*cos(th1 + th2 + th3 + th4))/2 + (gravi*l3*m3*cos(th1 + th2 + th3))/2 + gravi*l3*m4*cos(th1 + th2 + th3) + (dth1^2*l1*l3*m3*sin(th2 + th3))/2 + dth1^2*l1*l3*m4*sin(th2 + th3) + (dth1^2*l2*l4*m4*sin(th3 + th4))/2 + (dth2^2*l2*l4*m4*sin(th3 + th4))/2 + (dth1^2*l2*l3*m3*sin(th3))/2 + dth1^2*l2*l3*m4*sin(th3) + (dth2^2*l2*l3*m3*sin(th3))/2 + dth2^2*l2*l3*m4*sin(th3) - (dth4^2*l3*l4*m4*sin(th4))/2 + (dth1^2*l1*l4*m4*sin(th2 + th3 + th4))/2 + dth1*dth2*l2*l4*m4*sin(th3 + th4) + dth1*dth2*l2*l3*m3*sin(th3) + 2*dth1*dth2*l2*l3*m4*sin(th3) - dth1*dth4*l3*l4*m4*sin(th4) - dth2*dth4*l3*l4*m4*sin(th4) - dth3*dth4*l3*l4*m4*sin(th4); ((l4*m4*cos(th1 + th2 + th3 + th4))/2)*gravi + (l4*m4*(dth1^2*l2*sin(th3 + th4) + dth2^2*l2*sin(th3 + th4) + dth1^2*l3*sin(th4) + dth2^2*l3*sin(th4) + dth3^2*l3*sin(th4) + dth1^2*l1*sin(th2 + th3 + th4) + 2*dth1*dth2*l2*sin(th3 + th4) + 2*dth1*dth2*l3*sin(th4) + 2*dth1*dth3*l3*sin(th4) + 2*dth2*dth3*l3*sin(th4)))/2; ((l5*m5*cos(th1 + th2 + th5))/2)*gravi + (l5*m5*(dth1^2*l1*sin(th2 + th5) + dth1^2*l2*sin(th5) + dth2^2*l2*sin(th5) + 2*dth1*dth2*l2*sin(th5)))/2];

%% input torques mapping matrix
S = [
    0,0,0,0,0;
    0,0,0,0,0;
    1,0,0,0,0;
    0,1,0,0,0;
    0,0,1,0,0;
    0,0,0,1,0;
    0,0,-1,0,1;];

%% Single stance constraint Jacobian

J_c_x = [1, 0, 0, 0, 0, 0, 0];
dJ_c_x = [0, 0, 0, 0, 0, 0, 0];

J_c_y = [0, 1, 0, 0, 0, 0, 0];

J_c_SS = [J_c_x; J_c_y];

%% Biarticular Spring Force

% Calculating the knee and hip angles
% We meed wrapTo2Pi() because some angles increase to inf due to the reset
% function eg. th1 and th5

phi_h_st = mod(th5 - pi, 2*pi); % angle between torso and stance thigh
phi_k_st = mod(pi - th2, 2*pi); % angle between stance thigh and shank
phi_h_sw = mod(th5 - th3, 2*pi); % angle between torso and swing thigh
phi_k_sw = mod(th4 - pi, 2*pi); % angle between swing thigh and shank

% Calculating the elongation in the springs
delta_l_st = r_h*(phi_h_st - phi_h0) - r_k*(phi_k_st - phi_k0); % elongation of BA in stance leg [m]
delta_l_sw = r_h*(phi_h_sw - phi_h0) - r_k*(phi_k_sw - phi_k0); % elongation of BA in swing leg [m]

% torques due to BA in stance leg
tau_st = [
    0;
    0;
    0;
    -k_ba*delta_l_st*r_k;
    0;
    0;
    -k_ba*delta_l_st*r_h];

% torques due to BA in swing leg
tau_sw = [
    0;
    0;
    0;
    0;
    k_ba*delta_l_sw*r_h;
    k_ba*delta_l_sw*r_k;
    -k_ba*delta_l_sw*r_h];

tau = tau_st + tau_sw;

%% Calculate the ground reaction force
lambda_y = max(k_ground*(y_ground_curr - y_st), 0) - d_ground*dy_st;
lambda_x = -inv(J_c_x*inv(MM)*J_c_x')*(J_c_x*inv(MM)*(S*U + tau +J_c_y'*lambda_y- HH)+dJ_c_x*dq);

lambda = [lambda_x; lambda_y];
%% Acceleration Calculation
ddq = inv(MM)*(- HH + S*U + tau + transpose(J_c_SS)*lambda);

%%
dX = [dq; ddq];

end

== matlab function model_5LinkWalk_NODS_soft_ground/Feedback_ff_controller/Feedback_ff_controller ==
  settings: updateMethod=DISCRETE
  data: t input; X input; U output; des_theta output; des_theta_alpha output; flag_des_theta_not_defined output; param input; joint_angles_ref input; landing_ref input; gains input; flag input
function [U, des_theta, des_theta_alpha, flag_des_theta_not_defined] = fcn(t, X, param, joint_angles_ref, landing_ref, gains,  flag)
coder.extrinsic('quadprog');
coder.extrinsic('sparse')

%% variables (absolute angles)
x_st = X(1);
y_st = X(2);
th1 = X(3);
th2 = X(4);
th3 = X(5);
th4 = X(6);
th5 = X(7);

dx_st = X(8);
dy_st = X(9);
dth1 = X(10);
dth2 = X(11);
dth3 = X(12);
dth4 = X(13);
dth5 = X(14);

q_non_floating = [th1;th2;th3;th4;th5];
dq_non_floating = [dth1;dth2;dth3;dth4;dth5];

%% Parameters

m1 = param(1);
m2 = param(2);
m3 = m2;
m4 = m1;
m5 = param(3);

l1 = param(4);
l2 = param(5);
l5 = param(6);
l3 = l2;
l4 = l1;

gravi = param(7);
I1 = param(8);
I2 = param(9);
I5 = param(10);
I3 = I1;
I4 = I2;

r_k = param(11);
r_h = param(12);
k_ba = param(13);
phi_h0 = param(14);
phi_k0 = param(15);

%% flags
f_impact = flag(1); % indicates which stance phase it is
foot = flag(2); % location of the stance foot
foot_prev = flag(3); % previous location of the stance foot
t_mode_change = flag(4); % time stamp when the mode change happens (TD or LO)
alpha_TD = flag(5); % lift off location of CoM when it happened
f_alpha_ob = flag(6); % alpha is out of bounds flag

%% Inertia Matrix
MM = MM_matrix([q_non_floating; dq_non_floating],param);

%% Centrifugal force · Coriolis force Vector
CC = zeros(5,1);

CC(1, 1) = - (dth2^2*l1*l3*m3*sin(th2 + th3))/2 - dth2^2*l1*l3*m4*sin(th2 + th3) - (dth3^2*l1*l3*m3*sin(th2 + th3))/2 - dth3^2*l1*l3*m4*sin(th2 + th3) - (dth2^2*l1*l5*m5*sin(th2 + th5))/2 - (dth3^2*l2*l4*m4*sin(th3 + th4))/2 - (dth4^2*l2*l4*m4*sin(th3 + th4))/2 - (dth5^2*l1*l5*m5*sin(th2 + th5))/2 - (dth2^2*l1*l2*m2*sin(th2))/2 - dth2^2*l1*l2*m3*sin(th2) - dth2^2*l1*l2*m4*sin(th2) - dth2^2*l1*l2*m5*sin(th2) - (dth3^2*l2*l3*m3*sin(th3))/2 - dth3^2*l2*l3*m4*sin(th3) - (dth4^2*l3*l4*m4*sin(th4))/2 - (dth5^2*l2*l5*m5*sin(th5))/2 - (dth2^2*l1*l4*m4*sin(th2 + th3 + th4))/2 - (dth3^2*l1*l4*m4*sin(th2 + th3 + th4))/2 - (dth4^2*l1*l4*m4*sin(th2 + th3 + th4))/2 - dth1*dth2*l1*l3*m3*sin(th2 + th3) - 2*dth1*dth2*l1*l3*m4*sin(th2 + th3) - dth1*dth3*l1*l3*m3*sin(th2 + th3) - 2*dth1*dth3*l1*l3*m4*sin(th2 + th3) - dth2*dth3*l1*l3*m3*sin(th2 + th3) - 2*dth2*dth3*l1*l3*m4*sin(th2 + th3) - dth1*dth2*l1*l5*m5*sin(th2 + th5) - dth1*dth3*l2*l4*m4*sin(th3 + th4) - dth1*dth4*l2*l4*m4*sin(th3 + th4) - dth2*dth3*l2*l4*m4*sin(th3 + th4) - dth2*dth4*l2*l4*m4*sin(th3 + th4) - dth1*dth5*l1*l5*m5*sin(th2 + th5) - dth3*dth4*l2*l4*m4*sin(th3 + th4) - dth2*dth5*l1*l5*m5*sin(th2 + th5) - dth1*dth2*l1*l2*m2*sin(th2) - 2*dth1*dth2*l1*l2*m3*sin(th2) - 2*dth1*dth2*l1*l2*m4*sin(th2) - 2*dth1*dth2*l1*l2*m5*sin(th2) - dth1*dth3*l2*l3*m3*sin(th3) - 2*dth1*dth3*l2*l3*m4*sin(th3) - dth2*dth3*l2*l3*m3*sin(th3) - 2*dth2*dth3*l2*l3*m4*sin(th3) - dth1*dth4*l3*l4*m4*sin(th4) - dth2*dth4*l3*l4*m4*sin(th4) - dth3*dth4*l3*l4*m4*sin(th4) - dth1*dth5*l2*l5*m5*sin(th5) - dth2*dth5*l2*l5*m5*sin(th5) - dth1*dth2*l1*l4*m4*sin(th2 + th3 + th4) - dth1*dth3*l1*l4*m4*sin(th2 + th3 + th4) - dth1*dth4*l1*l4*m4*sin(th2 + th3 + th4) - dth2*dth3*l1*l4*m4*sin(th2 + th3 + th4) - dth2*dth4*l1*l4*m4*sin(th2 + th3 + th4) - dth3*dth4*l1*l4*m4*sin(th2 + th3 + th4);
CC(2, 1) = (dth1^2*l1*l3*m3*sin(th2 + th3))/2 + dth1^2*l1*l3*m4*sin(th2 + th3) + (dth1^2*l1*l5*m5*sin(th2 + th5))/2 - (dth3^2*l2*l4*m4*sin(th3 + th4))/2 - (dth4^2*l2*l4*m4*sin(th3 + th4))/2 + (dth1^2*l1*l2*m2*sin(th2))/2 + dth1^2*l1*l2*m3*sin(th2) + dth1^2*l1*l2*m4*sin(th2) + dth1^2*l1*l2*m5*sin(th2) - (dth3^2*l2*l3*m3*sin(th3))/2 - dth3^2*l2*l3*m4*sin(th3) - (dth4^2*l3*l4*m4*sin(th4))/2 - (dth5^2*l2*l5*m5*sin(th5))/2 + (dth1^2*l1*l4*m4*sin(th2 + th3 + th4))/2 - dth1*dth3*l2*l4*m4*sin(th3 + th4) - dth1*dth4*l2*l4*m4*sin(th3 + th4) - dth2*dth3*l2*l4*m4*sin(th3 + th4) - dth2*dth4*l2*l4*m4*sin(th3 + th4) - dth3*dth4*l2*l4*m4*sin(th3 + th4) - dth1*dth3*l2*l3*m3*sin(th3) - 2*dth1*dth3*l2*l3*m4*sin(th3) - dth2*dth3*l2*l3*m3*sin(th3) - 2*dth2*dth3*l2*l3*m4*sin(th3) - dth1*dth4*l3*l4*m4*sin(th4) - dth2*dth4*l3*l4*m4*sin(th4) - dth3*dth4*l3*l4*m4*sin(th4) - dth1*dth5*l2*l5*m5*sin(th5) - dth2*dth5*l2*l5*m5*sin(th5);
CC(3, 1) = (dth1^2*l1*l3*m3*sin(th2 + th3))/2 + dth1^2*l1*l3*m4*sin(th2 + th3) + (dth1^2*l2*l4*m4*sin(th3 + th4))/2 + (dth2^2*l2*l4*m4*sin(th3 + th4))/2 + (dth1^2*l2*l3*m3*sin(th3))/2 + dth1^2*l2*l3*m4*sin(th3) + (dth2^2*l2*l3*m3*sin(th3))/2 + dth2^2*l2*l3*m4*sin(th3) - (dth4^2*l3*l4*m4*sin(th4))/2 + (dth1^2*l1*l4*m4*sin(th2 + th3 + th4))/2 + dth1*dth2*l2*l4*m4*sin(th3 + th4) + dth1*dth2*l2*l3*m3*sin(th3) + 2*dth1*dth2*l2*l3*m4*sin(th3) - dth1*dth4*l3*l4*m4*sin(th4) - dth2*dth4*l3*l4*m4*sin(th4) - dth3*dth4*l3*l4*m4*sin(th4);
CC(4, 1) = (l4*m4*(dth1^2*l2*sin(th3 + th4) + dth2^2*l2*sin(th3 + th4) + dth1^2*l3*sin(th4) + dth2^2*l3*sin(th4) + dth3^2*l3*sin(th4) + dth1^2*l1*sin(th2 + th3 + th4) + 2*dth1*dth2*l2*sin(th3 + th4) + 2*dth1*dth2*l3*sin(th4) + 2*dth1*dth3*l3*sin(th4) + 2*dth2*dth3*l3*sin(th4)))/2;
CC(5, 1) = (l5*m5*(dth1^2*l1*sin(th2 + th5) + dth1^2*l2*sin(th5) + dth2^2*l2*sin(th5) + 2*dth1*dth2*l2*sin(th5)))/2;

%% Gravity Vector
GG = zeros(5,1);

GG(1, 1) = (m3*(l2*cos(th1 + th2) + l1*cos(th1) + (l3*cos(th1 + th2 + th3))/2) + m5*(l2*cos(th1 + th2) + l1*cos(th1) + (l5*cos(th1 + th2 + th5))/2) + m2*((l2*cos(th1 + th2))/2 + l1*cos(th1)) + m4*((l4*cos(th1 + th2 + th3 + th4))/2 + l2*cos(th1 + th2) + l1*cos(th1) + l3*cos(th1 + th2 + th3)) + (l1*m1*cos(th1))/2)*gravi;
GG(2, 1) = (m3*(l2*cos(th1 + th2) + (l3*cos(th1 + th2 + th3))/2) + m5*(l2*cos(th1 + th2) + (l5*cos(th1 + th2 + th5))/2) + m4*((l4*cos(th1 + th2 + th3 + th4))/2 + l2*cos(th1 + th2) + l3*cos(th1 + th2 + th3)) + (l2*m2*cos(th1 + th2))/2)*gravi;
GG(3, 1) = (m4*((l4*cos(th1 + th2 + th3 + th4))/2 + l3*cos(th1 + th2 + th3)) + (l3*m3*cos(th1 + th2 + th3))/2)*gravi;
GG(4, 1) = ((l4*m4*cos(th1 + th2 + th3 + th4))/2)*gravi;
GG(5, 1) = ((l5*m5*cos(th1 + th2 + th5))/2)*gravi;

%% input torques mapping matrix
S = [
    0,0,0,0;
    1,0,0,0;
    0,1,0,0;
    0,0,1,0;
    0,-1,0,1;];

%% Calculating the biarticular muscle torques

% Calculating the knee and hip angles
% We meed wrapTo2Pi() because some angles increase to inf due to the reset
% function eg. th1 and th5. here also X(i) is used because i usually used
% relative angles for this calculation.

phi_h_st = mod(th5 - pi, 2*pi); % angle between torso and stance thigh
phi_k_st = mod(pi - th2, 2*pi); % angle between stance thigh and shank
phi_h_sw = mod(th5 - th3, 2*pi); % angle between torso and swing thigh
phi_k_sw = mod(th4 - pi,2 *pi); % angle between swing thigh and shank

% Calculating the elongation in the springs
delta_l_st = r_h*(phi_h_st - phi_h0) - r_k*(phi_k_st - phi_k0); % elongation of BA in stance leg [m]
delta_l_sw = r_h*(phi_h_sw - phi_h0) - r_k*(phi_k_sw - phi_k0); % elongation of BA in swing leg [m]

% torques due to BA in stance leg
tau_st = [
    0;
    -k_ba*delta_l_st*r_k;
    0;
    0;
    -k_ba*delta_l_st*r_h];

% torques due to BA in swing leg
tau_sw = [
    0;
    0;
    k_ba*delta_l_sw*r_h;
    k_ba*delta_l_sw*r_k;
    -k_ba*delta_l_sw*r_h];

%% Trajectories from OpenOCL
time_ref = joint_angles_ref(:,1);

th1_ref = joint_angles_ref(:,2);
th2_ref = joint_angles_ref(:,3);
th3_ref = joint_angles_ref(:,4);
th4_ref = joint_angles_ref(:,5);
th5_ref = joint_angles_ref(:,6);

dth1_ref = joint_angles_ref(:,7);
dth2_ref = joint_angles_ref(:,8);
dth3_ref = joint_angles_ref(:,9);
dth4_ref = joint_angles_ref(:,10);
dth5_ref = joint_angles_ref(:,11);

alpha_ref = joint_angles_ref(:,12);

t_curr_step = t - t_mode_change; % timer for the current step, relative to the LO or TD time

alpha = pi - (2*th1 + th2)/2;

if t_curr_step <= time_ref(end)
    % if the current time is within the ref. traj. time
    
    th1_des = interp1(time_ref, th1_ref, t_curr_step);
    th2_des = interp1(time_ref, th2_ref, t_curr_step);
    th3_des = interp1(time_ref, th3_ref, t_curr_step);
    th4_des = interp1(time_ref, th4_ref, t_curr_step);
    th5_des = interp1(time_ref, th5_ref, t_curr_step);
    
    dth1_des = interp1(time_ref, dth1_ref, t_curr_step);
    dth2_des = interp1(time_ref, dth2_ref, t_curr_step);
    dth3_des = interp1(time_ref, dth3_ref, t_curr_step);
    dth4_des = interp1(time_ref, dth4_ref, t_curr_step);
    dth5_des = interp1(time_ref, dth5_ref, t_curr_step);
else
    % if the current time has passed the ref. traj. time
    
    th1_des = th1_ref(end);
    th2_des = th2_ref(end);
    th3_des = th3_ref(end);
    th4_des = th4_ref(end);
    th5_des = th5_ref(end);
    
    dth1_des = dth1;
    dth2_des = dth2;
    dth3_des = dth3;
    dth4_des = dth4;
    dth5_des = dth5;
end

%% prev alpha is out of bounds controller v1
flag_landing = 0; % to check when the landing reference is activated

if f_alpha_ob == 0
    % reference wrt virtual stance leg angle alpha
    th1_des_alpha = interp1(alpha_ref, th1_ref, alpha);
    th2_des_alpha = interp1(alpha_ref, th2_ref, alpha);
    th3_des_alpha = interp1(alpha_ref, th3_ref, alpha);
    th4_des_alpha = interp1(alpha_ref, th4_ref, alpha);
    th5_des_alpha = interp1(alpha_ref, th5_ref, alpha);
    
    dth1_des_alpha = interp1(alpha_ref, dth1_ref, alpha);
    dth2_des_alpha = interp1(alpha_ref, dth2_ref, alpha);
    dth3_des_alpha = interp1(alpha_ref, dth3_ref, alpha);
    dth4_des_alpha = interp1(alpha_ref, dth4_ref, alpha);
    dth5_des_alpha = interp1(alpha_ref, dth5_ref, alpha);
    
    if alpha > alpha_ref(end)
        
        %%%%%% landing ref
        %%%%%% %%%%%%%%%%%%%%%%%%%%%%%%%%%%%%%%%%%%%%%%%%%%%%%%%
        flag_landing = 1;
        
        th1_ref_landing = landing_ref(:,2);
        th2_ref_landing = landing_ref(:,3);
        th3_ref_landing = landing_ref(:,4);
        th4_ref_landing = landing_ref(:,5);
        th5_ref_landing = landing_ref(:,6);
        
        dth1_ref_landing = landing_ref(:,7);
        dth2_ref_landing = landing_ref(:,8);
        dth3_ref_landing = landing_ref(:,9);
        dth4_ref_landing = landing_ref(:,10);
        dth5_ref_landing = landing_ref(:,11);
        
        alpha_ref_landing = landing_ref(:,12);
        
        th1_des_alpha = interp1(alpha_ref_landing, th1_ref_landing, alpha);
        th2_des_alpha = interp1(alpha_ref_landing, th2_ref_landing, alpha);
        th3_des_alpha = interp1(alpha_ref_landing, th3_ref_landing, alpha);
        th4_des_alpha = interp1(alpha_ref_landing, th4_ref_landing, alpha);
        th5_des_alpha = interp1(alpha_ref_landing, th5_ref_landing, alpha);
        
        dth1_des_alpha = interp1(alpha_ref_landing, dth1_ref_landing, alpha);
        dth2_des_alpha = interp1(alpha_ref_landing, dth2_ref_landing, alpha);
        dth3_des_alpha = interp1(alpha_ref_landing, dth3_ref_landing, alpha);
        dth4_des_alpha = interp1(alpha_ref_landing, dth4_ref_landing, alpha);
        dth5_des_alpha = interp1(alpha_ref_landing, dth5_ref_landing, alpha);
        %%%%%%%%%%%%%%%%%%%%%%%%%%%%%%%%%%%%%%%%%%%%%%%%%%%%%%%%%%%%
    end
    
else
    % f_alpha_ob == 1
    alpha_merge = alpha_ref(12); % alpha when the modified alpha should merge with alpha
    
    if alpha < alpha_merge
        a = (alpha_ref(1) - alpha_TD)/(alpha_TD - alpha_merge);
        b = -a*alpha_merge;
        
        alpha_mod = alpha + a*alpha + b;
        
        % sometimes modified alpha can be slightly smaller than alpha*(0)
        if alpha_mod < alpha_ref(1)
            alpha_mod = alpha_ref(1);
        end
        
        th1_des_alpha = interp1(alpha_ref, th1_ref, alpha_mod);
        th2_des_alpha = interp1(alpha_ref, th2_ref, alpha_mod);
        th3_des_alpha = interp1(alpha_ref, th3_ref, alpha_mod);
        th4_des_alpha = interp1(alpha_ref, th4_ref, alpha_mod);
        th5_des_alpha = interp1(alpha_ref, th5_ref, alpha_mod);
        
        dth1_des_alpha = interp1(alpha_ref, dth1_ref, alpha_mod);
        dth2_des_alpha = interp1(alpha_ref, dth2_ref, alpha_mod);
        dth3_des_alpha = interp1(alpha_ref, dth3_ref, alpha_mod);
        dth4_des_alpha = interp1(alpha_ref, dth4_ref, alpha_mod);
        dth5_des_alpha = interp1(alpha_ref, dth5_ref, alpha_mod);
        
    elseif alpha <= alpha_ref(end)
        th1_des_alpha = interp1(alpha_ref, th1_ref, alpha);
        th2_des_alpha = interp1(alpha_ref, th2_ref, alpha);
        th3_des_alpha = interp1(alpha_ref, th3_ref, alpha);
        th4_des_alpha = interp1(alpha_ref, th4_ref, alpha);
        th5_des_alpha = interp1(alpha_ref, th5_ref, alpha);
        
        dth1_des_alpha = interp1(alpha_ref, dth1_ref, alpha);
        dth2_des_alpha = interp1(alpha_ref, dth2_ref, alpha);
        dth3_des_alpha = interp1(alpha_ref, dth3_ref, alpha);
        dth4_des_alpha = interp1(alpha_ref, dth4_ref, alpha);
        dth5_des_alpha = interp1(alpha_ref, dth5_ref, alpha);
        
    else
        % alpha > alpha_ref(end)

        
        %%%%%% landing ref
        %%%%%% %%%%%%%%%%%%%%%%%%%%%%%%%%%%%%%%%%%%%%%%%%%%%%%%%
        flag_landing = 1;
        
        th1_ref_landing = landing_ref(:,2);
        th2_ref_landing = landing_ref(:,3);
        th3_ref_landing = landing_ref(:,4);
        th4_ref_landing = landing_ref(:,5);
        th5_ref_landing = landing_ref(:,6);
        
        dth1_ref_landing = landing_ref(:,7);
        dth2_ref_landing = landing_ref(:,8);
        dth3_ref_landing = landing_ref(:,9);
        dth4_ref_landing = landing_ref(:,10);
        dth5_ref_landing = landing_ref(:,11);
        
        alpha_ref_landing = landing_ref(:,12);
        
        th1_des_alpha = interp1(alpha_ref_landing, th1_ref_landing, alpha);
        th2_des_alpha = interp1(alpha_ref_landing, th2_ref_landing, alpha);
        th3_des_alpha = interp1(alpha_ref_landing, th3_ref_landing, alpha);
        th4_des_alpha = interp1(alpha_ref_landing, th4_ref_landing, alpha);
        th5_des_alpha = interp1(alpha_ref_landing, th5_ref_landing, alpha);
        
        dth1_des_alpha = interp1(alpha_ref_landing, dth1_ref_landing, alpha);
        dth2_des_alpha = interp1(alpha_ref_landing, dth2_ref_landing, alpha);
        dth3_des_alpha = interp1(alpha_ref_landing, dth3_ref_landing, alpha);
        dth4_des_alpha = interp1(alpha_ref_landing, dth4_ref_landing, alpha);
        dth5_des_alpha = interp1(alpha_ref_landing, dth5_ref_landing, alpha);
        %%%%%%%%%%%%%%%%%%%%%%%%%%%%%%%%%%%%%%%%%%%%%%%%%%%%%%%%%%%%
    end    
end

%%
flag_des_theta_not_defined = 0;
if isnan(th1_des_alpha)
    flag_des_theta_not_defined = 1;
    K_P1 = gains(1); % gain for CoM control
    K_D1 = gains(2); % gain for CoM control
end


%% Controller Gains
K_P1 = gains(1); % gain for CoM control
K_D1 = gains(2); % gain for CoM control
K_P2 = gains(3); % gain for CoM control
K_D2 = gains(4); % gain for CoM control
K_P3 = gains(5); % gain for CoM control
K_D3 = gains(6); % gain for CoM control
K_P4 = gains(7); % gain for CoM control
K_D4 = gains(8); % gain for CoM control
K_P5 = gains(9); % gain for CoM control
K_D5 = gains(10); % gain for CoM control

%% Feedback linearization controller

% constant task space matrix
T = [
    0,1,0,0,0;
    0,0,1,0,0;
    0,0,0,1,0;
    0,0,0,0,1];

%% Output Feedback Control

%%%%% alpha ref %%%%%
y_alpha = [th2; th3; th4; th5] - [th2_des_alpha; th3_des_alpha; th4_des_alpha; th5_des_alpha];
dy_alpha = [dth2; dth3; dth4; dth5] - [dth2_des_alpha; dth3_des_alpha; dth4_des_alpha; dth5_des_alpha];

K_p = [
    K_P2, 0, 0, 0;
    0, K_P3, 0, 0;
    0, 0, K_P4, 0;
    0, 0, 0, K_P5];

K_d = [
    K_D2, 0, 0, 0;
    0, K_D3, 0, 0;
    0, 0, K_D4, 0;
    0, 0, 0, K_D5];

v_alpha = -K_p*y_alpha - K_d*dy_alpha;

% u_alpha_fb = inv(T*inv(MM)*S)*(v_alpha + T*inv(MM)*(CC+GG));

% controller with BA muscles
u_alpha_fb = inv(T*inv(MM)*S)*(v_alpha + T*inv(MM)*(CC+GG-tau_st-tau_sw));

% u_alpha_ff = [u2_des; u3_des; u4_des; u5_des];
%%%%%%%%%%%%%%%%%%%%%

U = zeros(5,1);

U(1) = 0;
U(2) = u_alpha_fb(1);
U(3) = u_alpha_fb(2);
U(4) = u_alpha_fb(3);
U(5) = u_alpha_fb(4);

U(1) = 0;
U(2) = sign(U(2))*min(abs(U(2)), 200);
U(3) = sign(U(3))*min(abs(U(3)), 200);
U(4) = sign(U(4))*min(abs(U(4)), 200);
U(5) = sign(U(5))*min(abs(U(5)), 200);

%%
des_theta = [th1_des; th2_des; th3_des; th4_des; th5_des; dth1_des; dth2_des; dth3_des; dth4_des; dth5_des];
des_theta_alpha = [th1_des_alpha; th2_des_alpha; th3_des_alpha; th4_des_alpha; th5_des_alpha;
    dth1_des_alpha; dth2_des_alpha; dth3_des_alpha; dth4_des_alpha; dth5_des_alpha; flag_landing];

end
